simulink model "lqrtest"  (R2017b)
settings: Solver=VariableStepAuto  StartTime=0.0  StopTime=20  RelTol=1e-3
libraries: powerlib_meascontrol x1
settings Model: Creator=sm  LastModifiedBy=nimaaghli
settings CodeAppCC: StateflowObjectComments=on

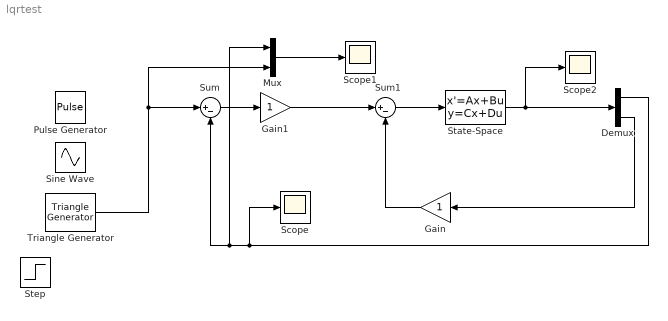
== system lqrtest ==
  Demux : Demux  Outputs=2
  Gain : Gain
  Gain1 : Gain
  Mux : Mux  Inputs=2
  Pulse Generator : DiscretePulseGenerator  PulseType=Time based  Period=10  PulseWidth=50
  Scope : Scope
  Scope1 : Scope
  Scope2 : Scope
  Sine Wave : Sin  SampleTime=0
  State-Space : StateSpace  A=[0,1;0,-1/0.1440]  B=[0;111.3292/0.1440]  C=[1,0;0,1]  D=[0;0]  InitialCondition=0
  Step : Step  SampleTime=0
  Sum : Sum  Inputs=|+-
  Sum1 : Sum  Inputs=|+-
  Triangle Generator : powerlib_meascontrol/Pulse & Signal Generators/Triangle Generator  Freq=20  Phase=90  Ts=0
  wires:
  State-Space/1 -> Scope2/1, Demux/1
  Sum/1 -> Gain1/1
  Demux/2 -> Gain/1
  Gain/1 -> Sum1/2
  Gain1/1 -> Sum1/1
  Sum1/1 -> State-Space/1
  Demux/1 -> Scope/1, Mux/1, Sum/2
  Mux/1 -> Scope1/1
  Triangle Generator/1 -> Sum/1, Mux/2
